simulink model "lumian"  (Simulink 8.3)
settings: Solver=ode45  StartTime=0.0  StopTime=1000.0  RelTol=1e-3
values from neighbouring files (symbols this model uses):
  K1 = 2*pi*n0*sqrt(gqn0*v)    [lumianzaihe.m]
  K2 = 2*pi*n00*v    (= 0.69115038379)    [lumianzaihe.m]
libraries: simulink x1
settings Model: Creator=xiagc  LastModifiedBy=USER
settings OptimizationCC: ExpressionDepthLimit=2147483647
settings DebuggingCC: FcnCallInpInsideContextMsg=UseLocalSettings

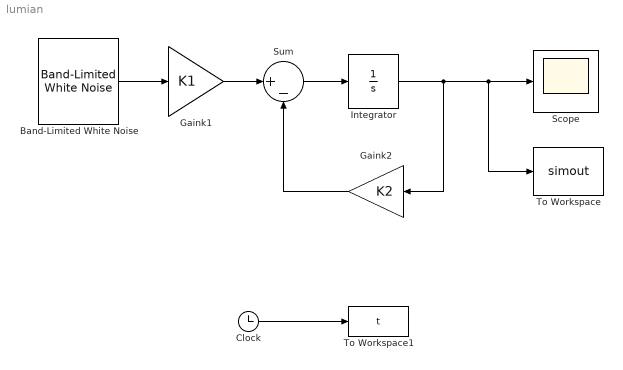
== system lumian ==
  Band-Limited White Noise : simulink/Sources/Band-Limited White Noise  Cov=1  Ts=0.001  seed=[23341]
  Clock : Clock
  Gaink1 : Gain  Gain=K1
  Gaink2 : Gain  Gain=K2
  Integrator : Integrator
  Scope : Scope
  Sum : Sum  Inputs=|+-
  To Workspace : ToWorkspace  VariableName=simout  SampleTime=-1
  To Workspace1 : ToWorkspace  VariableName=t  SampleTime=-1
  wires:
  Band-Limited White Noise/1 -> Gaink1/1
  Gaink1/1 -> Sum/1
  Integrator/1 -> Scope/1, To Workspace/1, Gaink2/1
  Sum/1 -> Integrator/1
  Gaink2/1 -> Sum/2
  Clock/1 -> To Workspace1/1
